simulink model "pottweitb"  (Simulink 8.5)
settings: Solver=ode45  SolverMode=SingleTasking  StartTime=0.0  StopTime=6  MaxStep=.002  RelTol=1e-3  AbsTol=1e-6
settings Model: Creator=PC  LastModifiedBy=PC  ExtModeTrigMode=oneshot  ExtModeArmWhenConnect=off
settings DataIOCC: LimitDataPoints=off
settings OptimizationCC: BlockReduction=off  BooleanDataType=off  ExpressionDepthLimit=128
settings DebuggingCC: SaveWithParameterizedLinksMsg=none  SignalResolutionControl=TryResolveAllWithWarning  MultiTaskDSMMsg=warning  MultiTaskCondExecSysMsg=none  FcnCallInpInsideContextMsg=EnableAllAsError  StateNameClashWarn=none  StrictBusMsg=None
settings HardwareCC: TargetUnknown=on

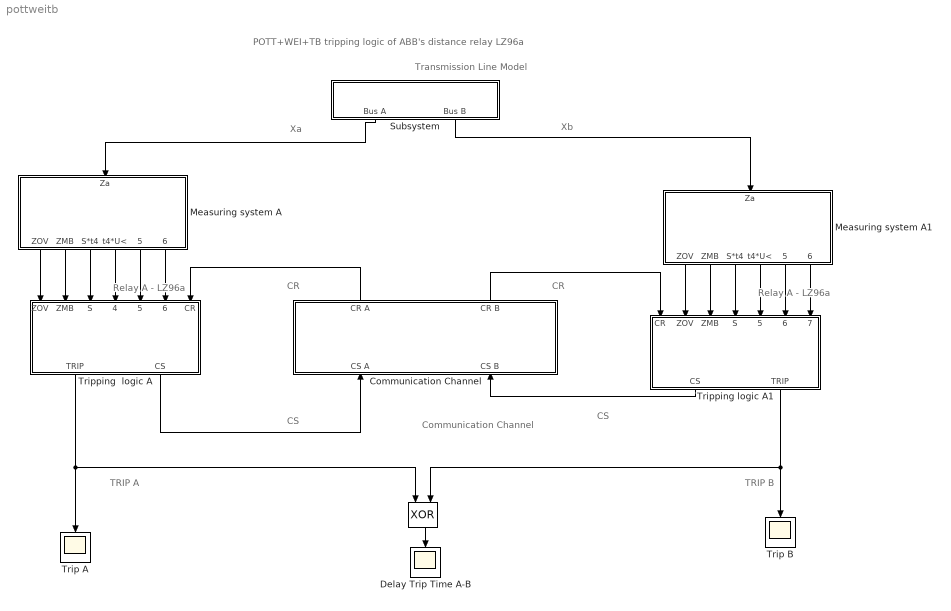
== system pottweitb ==
  note: Transmission Line Model
  note: Relay A - LZ96a
  note: Xa
  note: Xb
  note: CS
  note: CS
  note: CR
  note: CR
  note: TRIP A
  note: TRIP B
  note: POTT+WEI+TB tripping logic of ABB's distance relay LZ96a
  note: Communication
      | Channel
  note: Relay A - LZ96a
  " " : Logic  Operator=XOR
  Communication Channel : Subsystem  mask(Communication channel.){Tdelay=0, failureA=on, failureB=on, err_signal=0}
      mask prompts: Tdelay "Channel delay time [ms]:"; failureA "A to B Communication channel failure."; failureB "B to A Communication Channel failure"; err_signal "Erroneous signal:"
      mask TypeOptions err_signal: 0 | 1
  Delay Trip Time A-B : Scope
      settings: TickLabels=on  YMin=-0.5  YMax=2
  Measuring system A : Subsystem  mask(Measuring system - starter block){ZM=[1.4 1.7 2.7], Tzone=[0 0.5 1.0], S=[-1 3], Tstarter=1.5, ZMB=-1.5, UVR=[-1 2]}
      mask prompts: ZM "Zone reach [z1 z2  z3]  [p.u.]:"; Tzone "Zone times [z1 z2  z3]  [s]:"; S "Starter range [Smin Smax] [p.u.]:"; Tstarter "Starter time [s]:"; ZMB "ZMB (p.u.):"; UVR "undervoltage relay range [min max]"
      mask init:
      | ZM3=ZM(3);
      | ZM2=ZM(2);
      | ZOV=ZM(1);
      | t2=Tzone(2);
      | t3=Tzone(3);
      | t4=Tstarter;
      | s1=S(2);
      | s2=S(1);
      | ur=UVR(1);
      | ud=UVR(2);
  Measuring system A1 : Subsystem  mask(Measuring system - starter block){ZM=[1.4 1.7 2.7], Tzone=[0 0.5 1.0], S=[-1 3], Tstarter=1.5, ZMB=-1.5, UVR=[-1 2]}
      mask prompts: ZM "Zone reach [z1 z2  z3]  [p.u.]:"; Tzone "Zone times [z1 z2  z3]  [s]:"; S "Starter range [Smin Smax] [p.u.]:"; Tstarter "Starter time [s]:"; ZMB "ZMB (p.u.):"; UVR "undervoltage relay range [min max]"
      mask init:
      | ZM3=ZM(3);
      | ZM2=ZM(2);
      | ZOV=ZM(1);
      | t2=Tzone(2);
      | t3=Tzone(3);
      | t4=Tstarter;
      | s1=S(2);
      | s2=S(1);
      | ur=UVR(1);
      | ud=UVR(2);
  Subsystem : Subsystem  mask(Model of transmission line with fault){x=0.8, Tfault=2}
      mask prompts: x "Fault location from bus A [p.u.]"; Tfault "Fault time [s]:"
  Trip A : Scope
      settings: TickLabels=on  YMin=-0.5  YMax=2
  Trip B : Scope
      settings: TickLabels=on  YMin=-0.5  YMax=2
  Tripping  logic A : Subsystem  mask{tr=0.2}
      mask prompts: tr "Action Time of Relay"
  Tripping logic A1 : Subsystem  mask{tr=0.2}
      mask prompts: tr "Action Time of Relay"
  wires:
  " "/1 -> Delay Trip Time A-B/1
  Subsystem/1(Bus A) -> Measuring system A/1(Za)
  Measuring system A/6(ZM2*t2) -> Tripping  logic A/6(ZM2*t2)
  Measuring system A/5(ZM3*t3) -> Tripping  logic A/5(ZM3*t3)
  Measuring system A/4(t4*U<) -> Tripping  logic A/4(t4*U<)
  Measuring system A/3(S*t4) -> Tripping  logic A/3(S)
  Measuring system A/2(ZMB) -> Tripping  logic A/2(ZMB)
  Measuring system A/1(ZOV) -> Tripping  logic A/1(ZOV)
  Tripping  logic A/1(TRIP) -> Trip A/1, " "/1
  Tripping  logic A/2(CS) -> Communication Channel/1(CS A)
  Communication Channel/1(CR A) -> Tripping  logic A/7(CR)
  Measuring system A1/6(ZM2*t2) -> Tripping logic A1/7(ZM2*t2)
  Measuring system A1/5(ZM3*t3) -> Tripping logic A1/6(ZM3*t3)
  Measuring system A1/4(t4*U<) -> Tripping logic A1/5(t4*U<)
  Measuring system A1/3(S*t4) -> Tripping logic A1/4(S)
  Measuring system A1/2(ZMB) -> Tripping logic A1/3(ZMB)
  Measuring system A1/1(ZOV) -> Tripping logic A1/2(ZOV)
  Subsystem/2(Bus B) -> Measuring system A1/1(Za)
  Tripping logic A1/1(CS) -> Communication Channel/2(CS B)
  Tripping logic A1/2(TRIP) -> Trip B/1, " "/2
  Communication Channel/2(CR B) -> Tripping logic A1/1(CR)

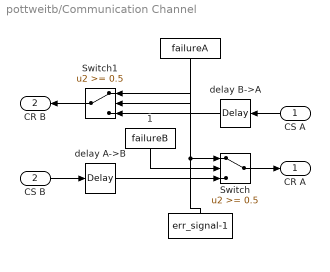
== system pottweitb/Communication Channel ==
  CS A : Inport
  CS B : Inport  Port=2
  " " : Constant  Value=failureA
  "  " : Constant  Value=err_signal-1
  " 1" : Constant  Value=failureB
  Switch : Switch  Threshold=0.5  SaturateOnIntegerOverflow=on  InputSameDT=on
  Switch1 : Switch  Threshold=0.5  SaturateOnIntegerOverflow=on  InputSameDT=on
  delay A->B : TransportDelay  DelayTime=Tdelay/1000+1e-12
  delay B->A : TransportDelay  DelayTime=Tdelay/1000+1e-12
  CR A : Outport  InitialOutput=0
  CR B : Outport  Port=2  InitialOutput=0
  wires:
  Switch/1 -> CR A/1
  CS B/1 -> delay A->B/1
  CS A/1 -> delay B->A/1
  Switch1/1 -> CR B/1
  "  "/1 -> Switch1/1, Switch/1
  delay A->B/1 -> Switch/3
  delay B->A/1 -> Switch1/3
  " "/1 -> Switch1/2
  " 1"/1 -> Switch/2

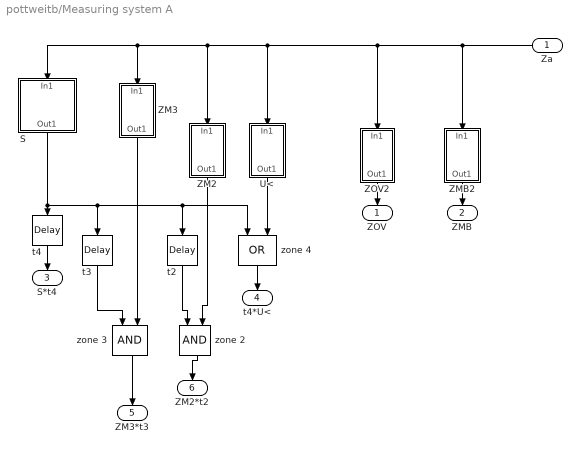
== system pottweitb/Measuring system A ==
  Za : Inport
  S : Subsystem  mask{s2=s2, s1=s1}
      mask prompts: s2 "starter (reverse side)"; s1 "starter (direct side)"
  U< : Subsystem  mask(undervoltage relay setting (reverse side)){ud=ud, ur=ur}
      mask prompts: ud "undervoltage relay (D)"; ur "undervoltage relay (R)"
  ZM2 : Subsystem  mask{ZM2=ZM2}
      mask prompts: ZM2 "zone 2"
  ZM3 : Subsystem  mask{ZM3=ZM3}
      mask prompts: ZM3 "zone 3"
  ZMB2 : Subsystem  mask{ZMB=ZMB}
      mask prompts: ZMB "MB"
  ZOV2 : Subsystem  mask{ZOV=ZOV}
      mask prompts: ZOV "zone 1"
  t2 : TransportDelay  DelayTime=t2
  t3 : TransportDelay  DelayTime=t3
  t4 : TransportDelay  DelayTime=t4
  zone 2 : Logic
  zone 3 : Logic
  zone 4 : Logic  Operator=OR
  ZOV : Outport
  ZMB : Outport  Port=2
  S*t4 : Outport  Port=3
  t4*U< : Outport  Port=4
  ZM3*t3 : Outport  Port=5
  ZM2*t2 : Outport  Port=6
  wires:
  Za/1 -> ZMB2/1(In1), ZOV2/1(In1), ZM2/1(In1), S/1(In1), ZM3/1(In1), U</1(In1)
  S/1(Out1) -> t4/1, t3/1, t2/1, zone 4/1
  t3/1 -> zone 3/1
  ZM3/1(Out1) -> zone 3/2
  t2/1 -> zone 2/1
  ZM2/1(Out1) -> zone 2/2
  U</1(Out1) -> zone 4/2
  ZOV2/1(Out1) -> ZOV/1
  ZMB2/1(Out1) -> ZMB/1
  t4/1 -> S*t4/1
  zone 4/1 -> t4*U</1
  zone 3/1 -> ZM3*t3/1
  zone 2/1 -> ZM2*t2/1

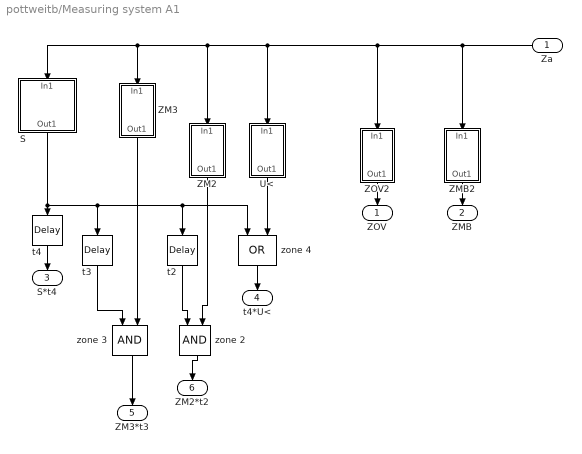
== system pottweitb/Measuring system A1 ==
  Za : Inport
  S : Subsystem  mask{s2=s2, s1=s1}
      mask prompts: s2 "starter (reverse side)"; s1 "starter (direct side)"
  U< : Subsystem  mask(undervoltage relay setting (reverse side)){ud=ud, ur=ur}
      mask prompts: ud "undervoltage relay (D)"; ur "undervoltage relay (R)"
  ZM2 : Subsystem  mask{ZM2=ZM2}
      mask prompts: ZM2 "zone 2"
  ZM3 : Subsystem  mask{ZM3=ZM3}
      mask prompts: ZM3 "zone 3"
  ZMB2 : Subsystem  mask{ZMB=ZMB}
      mask prompts: ZMB "MB"
  ZOV2 : Subsystem  mask{ZOV=ZOV}
      mask prompts: ZOV "zone 1"
  t2 : TransportDelay  DelayTime=t2
  t3 : TransportDelay  DelayTime=t3
  t4 : TransportDelay  DelayTime=t4
  zone 2 : Logic
  zone 3 : Logic
  zone 4 : Logic  Operator=OR
  ZOV : Outport
  ZMB : Outport  Port=2
  S*t4 : Outport  Port=3
  t4*U< : Outport  Port=4
  ZM3*t3 : Outport  Port=5
  ZM2*t2 : Outport  Port=6
  wires:
  zone 2/1 -> ZM2*t2/1
  zone 3/1 -> ZM3*t3/1
  zone 4/1 -> t4*U</1
  t4/1 -> S*t4/1
  ZMB2/1(Out1) -> ZMB/1
  ZOV2/1(Out1) -> ZOV/1
  U</1(Out1) -> zone 4/2
  ZM2/1(Out1) -> zone 2/2
  t2/1 -> zone 2/1
  ZM3/1(Out1) -> zone 3/2
  t3/1 -> zone 3/1
  S/1(Out1) -> zone 4/1, t2/1, t3/1, t4/1
  Za/1 -> U</1(In1), ZM3/1(In1), S/1(In1), ZM2/1(In1), ZOV2/1(In1), ZMB2/1(In1)

== system pottweitb/Subsystem ==
  (1-x) fault : Step  Time=Tfault  Before=1000  After=1-x  SampleTime=0
  x - fault : Step  Time=Tfault  Before=1000  After=x  SampleTime=0
  Bus A : Outport  InitialOutput=0
  Bus B : Outport  Port=2  InitialOutput=0
  wires:
  (1-x) fault/1 -> Bus B/1
  x - fault/1 -> Bus A/1

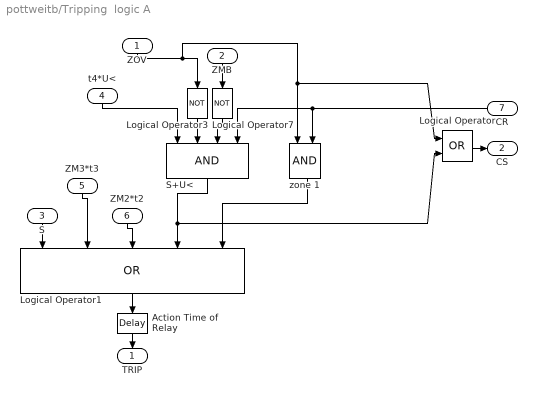
== system pottweitb/Tripping  logic A ==
  ZOV : Inport
  ZMB : Inport  Port=2
  S : Inport  Port=3
  t4*U< : Inport  Port=4
  ZM3*t3 : Inport  Port=5
  ZM2*t2 : Inport  Port=6
  CR : Inport  Port=7
  Action Time of Relay : TransportDelay  DelayTime=tr
  Logical Operator : Logic  Operator=OR
  Logical Operator1 : Logic  Operator=OR  Inputs=5
  Logical Operator3 : Logic  Operator=NOT  Inputs=1
  Logical Operator7 : Logic  Operator=NOT  Inputs=1
  S+U< : Logic  Inputs=4
  zone 1 : Logic
  TRIP : Outport  InitialOutput=0
  CS : Outport  Port=2
  wires:
  zone 1/1 -> Logical Operator1/5
  Action Time of Relay/1 -> TRIP/1
  Logical Operator/1 -> CS/1
  CR/1 -> zone 1/2, S+U</4
  Logical Operator7/1 -> S+U</3
  Logical Operator3/1 -> S+U</2
  Logical Operator1/1 -> Action Time of Relay/1
  S+U</1 -> Logical Operator1/4, Logical Operator/2
  ZMB/1 -> Logical Operator7/1
  t4*U</1 -> S+U</1
  ZM3*t3/1 -> Logical Operator1/2
  S/1 -> Logical Operator1/1
  ZM2*t2/1 -> Logical Operator1/3
  ZOV/1 -> Logical Operator3/1, zone 1/1, Logical Operator/1

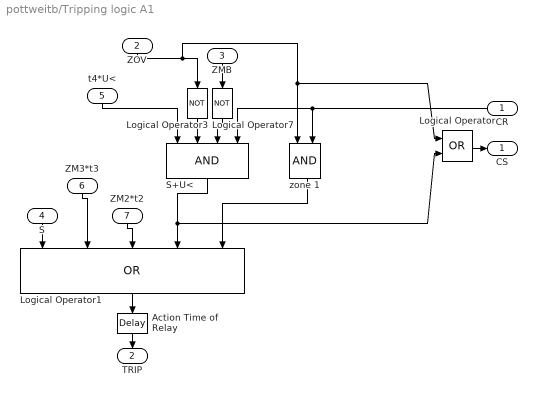
== system pottweitb/Tripping logic A1 ==
  CR : Inport
  ZOV : Inport  Port=2
  ZMB : Inport  Port=3
  S : Inport  Port=4
  t4*U< : Inport  Port=5
  ZM3*t3 : Inport  Port=6
  ZM2*t2 : Inport  Port=7
  Action Time of Relay : TransportDelay  DelayTime=tr
  Logical Operator : Logic  Operator=OR
  Logical Operator1 : Logic  Operator=OR  Inputs=5
  Logical Operator3 : Logic  Operator=NOT  Inputs=1
  Logical Operator7 : Logic  Operator=NOT  Inputs=1
  S+U< : Logic  Inputs=4
  zone 1 : Logic
  CS : Outport
  TRIP : Outport  Port=2  InitialOutput=0
  wires:
  zone 1/1 -> Logical Operator1/5
  Action Time of Relay/1 -> TRIP/1
  Logical Operator/1 -> CS/1
  CR/1 -> zone 1/2, S+U</4
  Logical Operator7/1 -> S+U</3
  Logical Operator3/1 -> S+U</2
  Logical Operator1/1 -> Action Time of Relay/1
  S+U</1 -> Logical Operator1/4, Logical Operator/2
  ZMB/1 -> Logical Operator7/1
  t4*U</1 -> S+U</1
  ZM3*t3/1 -> Logical Operator1/2
  S/1 -> Logical Operator1/1
  ZM2*t2/1 -> Logical Operator1/3
  ZOV/1 -> Logical Operator3/1, zone 1/1, Logical Operator/1

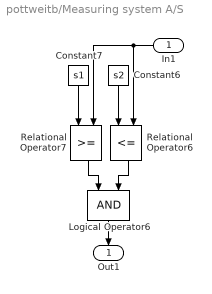
== system pottweitb/Measuring system A/S ==
  In1 : Inport
  Constant6 : Constant  Value=s2
  Constant7 : Constant  Value=s1
  Logical Operator6 : Logic
  Relational Operator6 : RelationalOperator  Operator=<=  InputSameDT=on
  Relational Operator7 : RelationalOperator  InputSameDT=on
  Out1 : Outport  InitialOutput=0
  wires:
  Constant6/1 -> Relational Operator6/1
  Constant7/1 -> Relational Operator7/1
  Relational Operator7/1 -> Logical Operator6/1
  Relational Operator6/1 -> Logical Operator6/2
  In1/1 -> Relational Operator6/2, Relational Operator7/2
  Logical Operator6/1 -> Out1/1

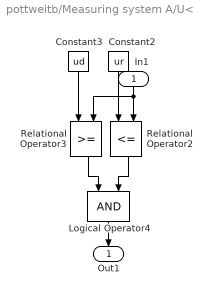
== system pottweitb/Measuring system A/U< ==
  In1 : Inport
  Constant2 : Constant  Value=ur
  Constant3 : Constant  Value=ud
  Logical Operator4 : Logic
  Relational Operator2 : RelationalOperator  Operator=<=  InputSameDT=on
  Relational Operator3 : RelationalOperator  InputSameDT=on
  Out1 : Outport  InitialOutput=0
  wires:
  Constant2/1 -> Relational Operator2/1
  Constant3/1 -> Relational Operator3/1
  Relational Operator3/1 -> Logical Operator4/1
  Relational Operator2/1 -> Logical Operator4/2
  Logical Operator4/1 -> Out1/1
  In1/1 -> Relational Operator2/2, Relational Operator3/2

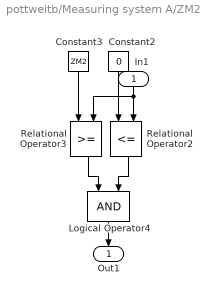
== system pottweitb/Measuring system A/ZM2 ==
  In1 : Inport
  Constant2 : Constant  Value=0
  Constant3 : Constant  Value=ZM2
  Logical Operator4 : Logic
  Relational Operator2 : RelationalOperator  Operator=<=  InputSameDT=on
  Relational Operator3 : RelationalOperator  InputSameDT=on
  Out1 : Outport  InitialOutput=0
  wires:
  Constant2/1 -> Relational Operator2/1
  Constant3/1 -> Relational Operator3/1
  Relational Operator3/1 -> Logical Operator4/1
  Relational Operator2/1 -> Logical Operator4/2
  Logical Operator4/1 -> Out1/1
  In1/1 -> Relational Operator2/2, Relational Operator3/2

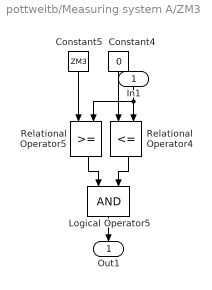
== system pottweitb/Measuring system A/ZM3 ==
  In1 : Inport
  Constant4 : Constant  Value=0
  Constant5 : Constant  Value=ZM3
  Logical Operator5 : Logic
  Relational Operator4 : RelationalOperator  Operator=<=  InputSameDT=on
  Relational Operator5 : RelationalOperator  InputSameDT=on
  Out1 : Outport  InitialOutput=0
  wires:
  Constant4/1 -> Relational Operator4/1
  Constant5/1 -> Relational Operator5/1
  Relational Operator5/1 -> Logical Operator5/1
  Relational Operator4/1 -> Logical Operator5/2
  Logical Operator5/1 -> Out1/1
  In1/1 -> Relational Operator4/2, Relational Operator5/2

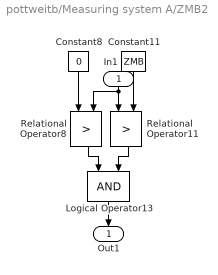
== system pottweitb/Measuring system A/ZMB2 ==
  In1 : Inport
  Constant11 : Constant  Value=ZMB
  Constant8 : Constant  Value=0
  Logical Operator13 : Logic
  Relational Operator11 : RelationalOperator  Operator=>  InputSameDT=on
  Relational Operator8 : RelationalOperator  Operator=>  InputSameDT=on
  Out1 : Outport  InitialOutput=0
  wires:
  Constant8/1 -> Relational Operator8/1
  Relational Operator8/1 -> Logical Operator13/1
  Relational Operator11/1 -> Logical Operator13/2
  Constant11/1 -> Relational Operator11/2
  Logical Operator13/1 -> Out1/1
  In1/1 -> Relational Operator11/1, Relational Operator8/2

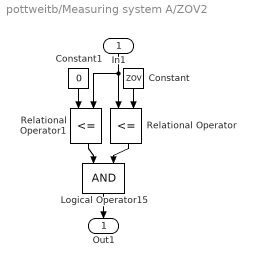
== system pottweitb/Measuring system A/ZOV2 ==
  In1 : Inport
  Constant : Constant  Value=ZOV
  Constant1 : Constant  Value=0
  Logical Operator15 : Logic
  Relational Operator : RelationalOperator  Operator=<=  InputSameDT=on
  Relational Operator1 : RelationalOperator  Operator=<=  InputSameDT=on
  Out1 : Outport  InitialOutput=0
  wires:
  In1/1 -> Relational Operator/1, Relational Operator1/2
  Constant/1 -> Relational Operator/2
  Constant1/1 -> Relational Operator1/1
  Relational Operator1/1 -> Logical Operator15/1
  Relational Operator/1 -> Logical Operator15/2
  Logical Operator15/1 -> Out1/1

== system pottweitb/Measuring system A1/S ==
  In1 : Inport
  Constant6 : Constant  Value=s2
  Constant7 : Constant  Value=s1
  Logical Operator6 : Logic
  Relational Operator6 : RelationalOperator  Operator=<=  InputSameDT=on
  Relational Operator7 : RelationalOperator  InputSameDT=on
  Out1 : Outport  InitialOutput=0
  wires:
  Logical Operator6/1 -> Out1/1
  In1/1 -> Relational Operator7/2, Relational Operator6/2
  Relational Operator6/1 -> Logical Operator6/2
  Relational Operator7/1 -> Logical Operator6/1
  Constant7/1 -> Relational Operator7/1
  Constant6/1 -> Relational Operator6/1

== system pottweitb/Measuring system A1/U< ==
  In1 : Inport
  Constant2 : Constant  Value=ur
  Constant3 : Constant  Value=ud
  Logical Operator4 : Logic
  Relational Operator2 : RelationalOperator  Operator=<=  InputSameDT=on
  Relational Operator3 : RelationalOperator  InputSameDT=on
  Out1 : Outport  InitialOutput=0
  wires:
  In1/1 -> Relational Operator3/2, Relational Operator2/2
  Logical Operator4/1 -> Out1/1
  Relational Operator2/1 -> Logical Operator4/2
  Relational Operator3/1 -> Logical Operator4/1
  Constant3/1 -> Relational Operator3/1
  Constant2/1 -> Relational Operator2/1

== system pottweitb/Measuring system A1/ZM2 ==
  In1 : Inport
  Constant2 : Constant  Value=0
  Constant3 : Constant  Value=ZM2
  Logical Operator4 : Logic
  Relational Operator2 : RelationalOperator  Operator=<=  InputSameDT=on
  Relational Operator3 : RelationalOperator  InputSameDT=on
  Out1 : Outport  InitialOutput=0
  wires:
  In1/1 -> Relational Operator3/2, Relational Operator2/2
  Logical Operator4/1 -> Out1/1
  Relational Operator2/1 -> Logical Operator4/2
  Relational Operator3/1 -> Logical Operator4/1
  Constant3/1 -> Relational Operator3/1
  Constant2/1 -> Relational Operator2/1

== system pottweitb/Measuring system A1/ZM3 ==
  In1 : Inport
  Constant4 : Constant  Value=0
  Constant5 : Constant  Value=ZM3
  Logical Operator5 : Logic
  Relational Operator4 : RelationalOperator  Operator=<=  InputSameDT=on
  Relational Operator5 : RelationalOperator  InputSameDT=on
  Out1 : Outport  InitialOutput=0
  wires:
  In1/1 -> Relational Operator5/2, Relational Operator4/2
  Logical Operator5/1 -> Out1/1
  Relational Operator4/1 -> Logical Operator5/2
  Relational Operator5/1 -> Logical Operator5/1
  Constant5/1 -> Relational Operator5/1
  Constant4/1 -> Relational Operator4/1

== system pottweitb/Measuring system A1/ZMB2 ==
  In1 : Inport
  Constant11 : Constant  Value=ZMB
  Constant8 : Constant  Value=0
  Logical Operator13 : Logic
  Relational Operator11 : RelationalOperator  Operator=>  InputSameDT=on
  Relational Operator8 : RelationalOperator  Operator=>  InputSameDT=on
  Out1 : Outport  InitialOutput=0
  wires:
  In1/1 -> Relational Operator8/2, Relational Operator11/1
  Logical Operator13/1 -> Out1/1
  Constant11/1 -> Relational Operator11/2
  Relational Operator11/1 -> Logical Operator13/2
  Relational Operator8/1 -> Logical Operator13/1
  Constant8/1 -> Relational Operator8/1

== system pottweitb/Measuring system A1/ZOV2 ==
  In1 : Inport
  Constant : Constant  Value=ZOV
  Constant1 : Constant  Value=0
  Logical Operator15 : Logic
  Relational Operator : RelationalOperator  Operator=<=  InputSameDT=on
  Relational Operator1 : RelationalOperator  Operator=<=  InputSameDT=on
  Out1 : Outport  InitialOutput=0
  wires:
  Logical Operator15/1 -> Out1/1
  Relational Operator/1 -> Logical Operator15/2
  Relational Operator1/1 -> Logical Operator15/1
  Constant1/1 -> Relational Operator1/1
  Constant/1 -> Relational Operator/2
  In1/1 -> Relational Operator1/2, Relational Operator/1
